simulink model "kupf"  (R2012a)
settings: Solver=ode45  SolverMode=SingleTasking  StartTime=0.0  StopTime=t_sym  RelTol=1e-3
settings Model: CovMetricSettings=dwe  CovHtmlReporting=off  covSaveCumulativeToWorkspaceVar=off  CovSaveSingleToWorkspaceVar=off  CovExternalEMLEnable=on  Creator=rafal  LastModifiedBy=rafal
settings DataIOCC: SaveFormat=StructureWithTime  ReturnWorkspaceOutputs=off
settings OptimizationCC: LifeSpan=inf  SimCompilerOptimization=Off
settings DebuggingCC: FcnCallInpInsideContextMsg=Enable All
settings HardwareCC: ProdWordSize=32  ProdHWDeviceType=Specified
settings SFSimCC: SimUseLocalCustomCode=off
settings RTWCC: RTWUseLocalCustomCode=off  RTWCompilerOptimization=Off
settings GRTTargetCC: CodeReplacementLibrary=C99 (ISO)  CPPClassGenCompliant=off

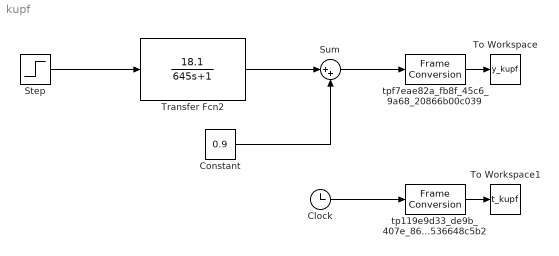
== system kupf ==
  Clock : Clock
  Constant : Constant  Value=0.9
  "Step " : Step  Time=235  SampleTime=0
  Sum : Sum  Inputs=|++
  To Workspace : ToWorkspace  VariableName=y_kupf  SampleTime=-1
  To Workspace1 : ToWorkspace  VariableName=t_kupf  SampleTime=-1
  Transfer Fcn2 : TransferFcn  Numerator=[18.1]  Denominator=[645 1]
  tp119e9d33_de9b_407e_864c_66536648c5b2 : FrameConversion  OutFrame=Sample-based
  tpf7eae82a_fb8f_45c6_9a68_20866b00c039 : FrameConversion  OutFrame=Sample-based
  wires:
  "Step "/1 -> Transfer Fcn2/1
  Transfer Fcn2/1 -> Sum/1
  Constant/1 -> Sum/2
  Sum/1 -> tpf7eae82a_fb8f_45c6_9a68_20866b00c039/1
  tpf7eae82a_fb8f_45c6_9a68_20866b00c039/1 -> To Workspace/1
  Clock/1 -> tp119e9d33_de9b_407e_864c_66536648c5b2/1
  tp119e9d33_de9b_407e_864c_66536648c5b2/1 -> To Workspace1/1
